simulink library "Hquad_control_LIB_MPC"  (Simulink 7.8)
settings: Solver=ode45  StartTime=0.0  StopTime=10.0  RelTol=1e-3
values from neighbouring files (symbols this model uses):
  FG_ctrl_x =     [kostas_malakies.mat]    (also in kostas_malakies2.mat)
  FG_ctrl_y =     [kostas_malakies.mat]    (also in kostas_malakies2.mat)
  FG_ctrl_yaw =     [kostas_malakies.mat]    (also in kostas_malakies2.mat)
  FG_ctrl_z =     [kostas_malakies.mat]    (also in kostas_malakies2.mat)
  g = 9.8065    [kostas_malakies.mat]    (also in kostas_malakies2.mat; load_PMModel.m = 9.81; main.m; main_last.m)
  kalm_mpc_x =     [kostas_malakies.mat]    (also in kostas_malakies2.mat)
  kalm_mpc_y =     [kostas_malakies.mat]    (also in kostas_malakies2.mat)
  kalm_mpc_yaw =     [kostas_malakies.mat]    (also in kostas_malakies2.mat)
  kalm_mpc_z =     [kostas_malakies.mat]    (also in kostas_malakies2.mat)
  MAX_BIAS_ANGLE = 0.0872664625997    [kostas_malakies.mat]    (also in kostas_malakies2.mat; main.m; main_last.m)
  MAX_BIAS_THRUST = 0.5    [kostas_malakies.mat]    (also in kostas_malakies2.mat; main.m; main_last.m)
  MAX_BIAS_YAW_RATE = 0.0872664625997    [kostas_malakies.mat]    (also in kostas_malakies2.mat; main.m; main_last.m)
  traj_FG =     [kostas.mat]    (also in kostas_malakies.mat; kostas_malakies2.mat; main_last.m = ReferenceCreator(maxdisty,maxdistz,scale_y,scale_z); traj_helix.mat)
  Ts = 0.02    [kostas_malakies.mat]    (also in kostas_malakies2.mat; main.m; main_last.m; matlab.mat = 0.08)
libraries: Hquad_control_LIB_MPC x17, simulink x9
(part 1 of 2)
settings Model: Creator=andi  LastModifiedBy=burrimi

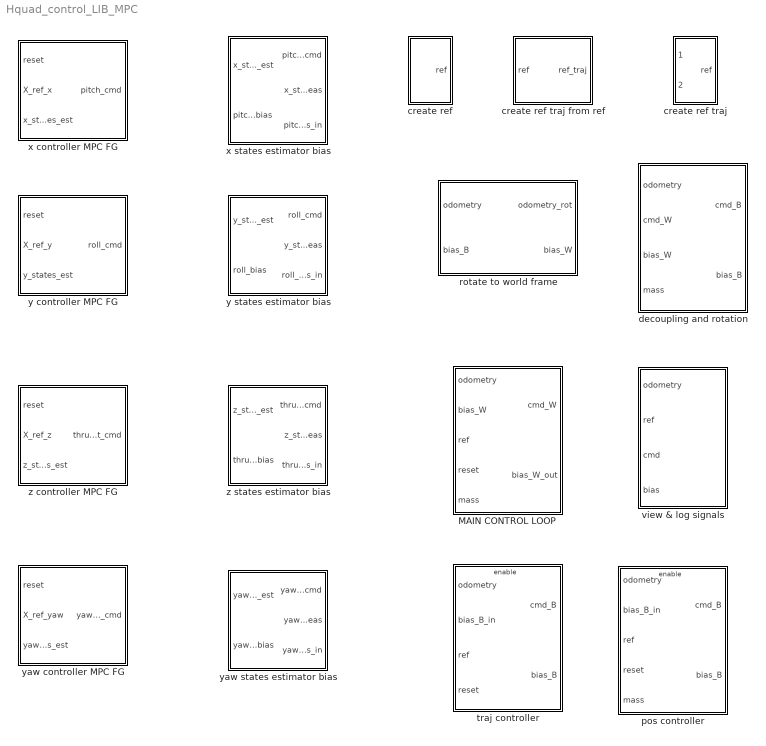
== system Hquad_control_LIB_MPC ==
  MAIN CONTROL LOOP : Subsystem  Priority=2  TreatAsAtomicUnit=on
  create ref : Subsystem
  create ref traj : Subsystem
  create ref traj from ref : Subsystem
  decoupling and rotation : Subsystem  Priority=3  TreatAsAtomicUnit=on
  pos controller : Subsystem
  rotate to world frame : Subsystem  Priority=1
  traj controller : Subsystem
  view & log signals : Subsystem
  "x controller MPC FG  " : Subsystem
  x states estimator bias : Subsystem
  y controller MPC FG : Subsystem
  y states estimator bias : Subsystem
  yaw controller MPC FG : Subsystem
  yaw states estimator bias : Subsystem
  z controller MPC FG : Subsystem
  z states estimator bias : Subsystem

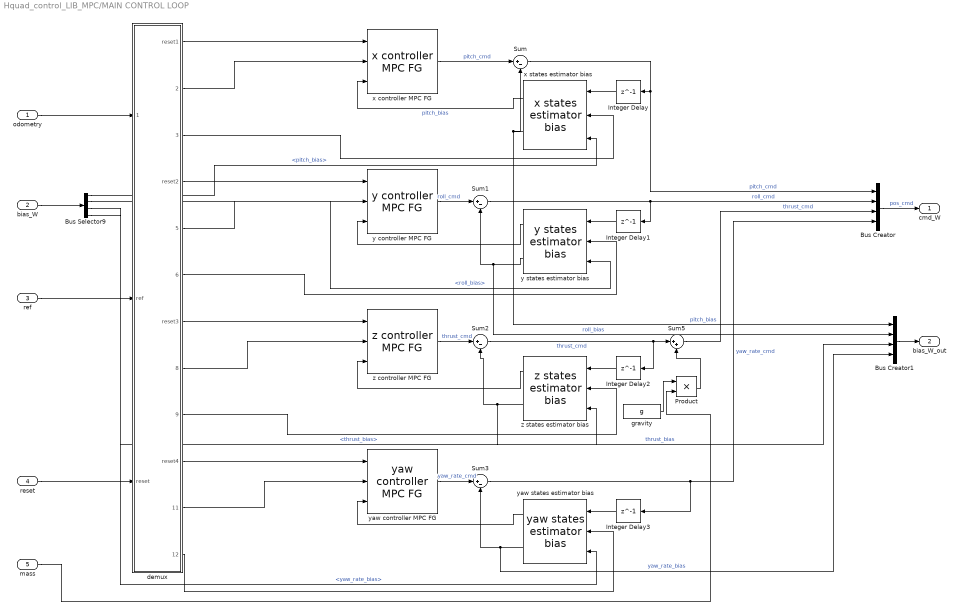
== system Hquad_control_LIB_MPC/MAIN CONTROL LOOP ==
  odometry : Inport
  bias_W : Inport  Port=2
  ref : Inport  Port=3
  reset : Inport  Port=4
  mass : Inport  Port=5
  Bus Creator : BusCreator
  Bus Creator1 : BusCreator
  Bus Selector9 : BusSelector  OutputSignals=pitch_bias,roll_bias,thrust_bias,yaw_rate_bias
  Integer Delay{,1..3} (4 alike) : Delay  DelayLength=1
  Product : Product  RndMeth=Zero
  Sum{,1..3} (4 alike) : Sum  Inputs=|+-
  Sum5 : Sum  Inputs=|++
  demux : Subsystem
  gravity : Constant  Value=g
  "x controller MPC FG  " : Hquad_control_LIB_MPC/x controller MPC FG  
  x states estimator bias : Hquad_control_LIB_MPC/x states estimator bias
  y controller MPC FG : Hquad_control_LIB_MPC/y controller MPC FG
  y states estimator bias : Hquad_control_LIB_MPC/y states estimator bias
  yaw controller MPC FG : Hquad_control_LIB_MPC/yaw controller MPC FG
  yaw states estimator bias : Hquad_control_LIB_MPC/yaw states estimator bias
  z controller MPC FG : Hquad_control_LIB_MPC/z controller MPC FG
  z states estimator bias : Hquad_control_LIB_MPC/z states estimator bias
  cmd_W : Outport
  bias_W_out : Outport  Port=2
  wires:
  gravity/1 -> Product/1
  Product/1 -> Sum5/2
  mass/1 -> Product/2
  demux/11(X_ref_yaw) -> yaw controller MPC FG/2
  demux/9(z_states_meas) -> z states estimator bias/2
  demux/6(y_states_meas) -> y states estimator bias/2
  demux/3(x_states_meas) -> x states estimator bias/2
  Bus Creator/1 -> cmd_W/1  "pos_cmd"
  demux/10(reset4) -> yaw controller MPC FG/1
  demux/7(reset3) -> z controller MPC FG/1
  demux/5(X_ref_y) -> y controller MPC FG/2
  demux/4(reset2) -> y controller MPC FG/1
  demux/1(reset1) -> "x controller MPC FG  "/1
  reset/1 -> demux/3(reset)
  ref/1 -> demux/2(ref)
  odometry/1 -> demux/1(odometry)
  Integer Delay2/1 -> z states estimator bias/1
  Integer Delay1/1 -> y states estimator bias/1
  demux/2(X_ref_x) -> "x controller MPC FG  "/2
  demux/8(X_ref_z) -> z controller MPC FG/2
  z states estimator bias/1 -> z controller MPC FG/3
  Integer Delay/1 -> x states estimator bias/1
  y states estimator bias/1 -> y controller MPC FG/3
  "x controller MPC FG  "/1 -> Sum/1  "pitch_cmd"
  Sum/1 -> Integer Delay/1, Bus Creator/1  "pitch_cmd"
  y controller MPC FG/1 -> Sum1/1  "roll_cmd"
  Sum1/1 -> Integer Delay1/1, Bus Creator/2  "roll_cmd"
  y states estimator bias/2 -> Sum1/2, Bus Creator1/2  "roll_bias"
  z states estimator bias/2 -> Sum2/2, Bus Creator1/3  "thrust_bias"
  z controller MPC FG/1 -> Sum2/1  "thrust_cmd"
  Sum2/1 -> Integer Delay2/1, Sum5/1  "thrust_cmd"
  Bus Creator1/1 -> bias_W_out/1
  Sum5/1 -> Bus Creator/3  "thrust_cmd"
  bias_W/1 -> Bus Selector9/1
  Bus Selector9/2 -> y states estimator bias/3  "<roll_bias>"
  Bus Selector9/1 -> x states estimator bias/3  "<pitch_bias>"
  demux/12(yaw_states_meas) -> yaw states estimator bias/2
  x states estimator bias/1 -> "x controller MPC FG  "/3  "pitch_bias"
  x states estimator bias/2 -> Bus Creator1/1, Sum/2  "pitch_bias"
  Bus Selector9/3 -> z states estimator bias/3  "<thrust_bias>"
  Integer Delay3/1 -> yaw states estimator bias/1
  yaw states estimator bias/1 -> yaw controller MPC FG/3
  yaw states estimator bias/2 -> Sum3/2, Bus Creator1/4  "yaw_rate_bias"
  yaw controller MPC FG/1 -> Sum3/1  "yaw_rate_cmd"
  Sum3/1 -> Bus Creator/4, Integer Delay3/1  "yaw_rate_cmd"
  Bus Selector9/4 -> yaw states estimator bias/3  "<yaw_rate_bias>"

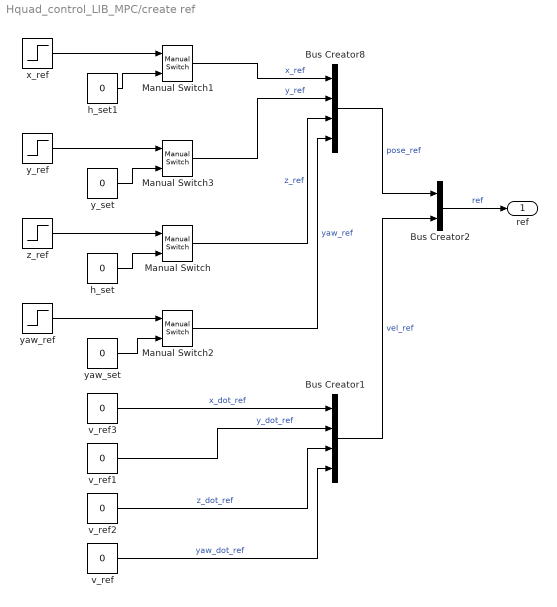
== system Hquad_control_LIB_MPC/create ref ==
  Bus Creator1 : BusCreator
  Bus Creator2 : BusCreator  Inputs=2
  Bus Creator8 : BusCreator
  Manual Switch{,1..3} (4 alike) : simulink/Signal Routing/Manual Switch  SystemSampleTime=-1  sw=1  action=0  varsize=off
  h_set : Constant  Value=0  OutDataTypeStr=double  SampleTime=-1
  h_set1 : Constant  Value=0  OutDataTypeStr=double  SampleTime=-1
  v_ref{,1..3} (4 alike) : Constant  Value=0  OutDataTypeStr=double  SampleTime=-1
  x_ref : Step  Time=5  SampleTime=0
  y_ref : Step  Time=15  SampleTime=0
  y_set : Constant  Value=0  OutDataTypeStr=double  SampleTime=-1
  yaw_ref : Step  Time=20  After=pi  SampleTime=0
  "yaw_set  " : Constant  Value=0  OutDataTypeStr=double  SampleTime=-1
  z_ref : Step  Time=15  SampleTime=0
  ref : Outport
  wires:
  yaw_ref/1 -> Manual Switch2/1
  "yaw_set  "/1 -> Manual Switch2/2
  h_set/1 -> Manual Switch/2
  z_ref/1 -> Manual Switch/1
  y_ref/1 -> Manual Switch3/1
  y_set/1 -> Manual Switch3/2
  h_set1/1 -> Manual Switch1/2
  Bus Creator2/1 -> ref/1  "ref"
  Bus Creator8/1 -> Bus Creator2/1  "pose_ref"
  Bus Creator1/1 -> Bus Creator2/2  "vel_ref"
  Manual Switch1/1 -> Bus Creator8/1  "x_ref"
  Manual Switch3/1 -> Bus Creator8/2  "y_ref"
  Manual Switch2/1 -> Bus Creator8/4  "yaw_ref"
  Manual Switch/1 -> Bus Creator8/3  "z_ref"
  v_ref/1 -> Bus Creator1/4  "yaw_dot_ref"
  v_ref3/1 -> Bus Creator1/1  "x_dot_ref"
  v_ref1/1 -> Bus Creator1/2  "y_dot_ref"
  v_ref2/1 -> Bus Creator1/3  "z_dot_ref"
  x_ref/1 -> Manual Switch1/1

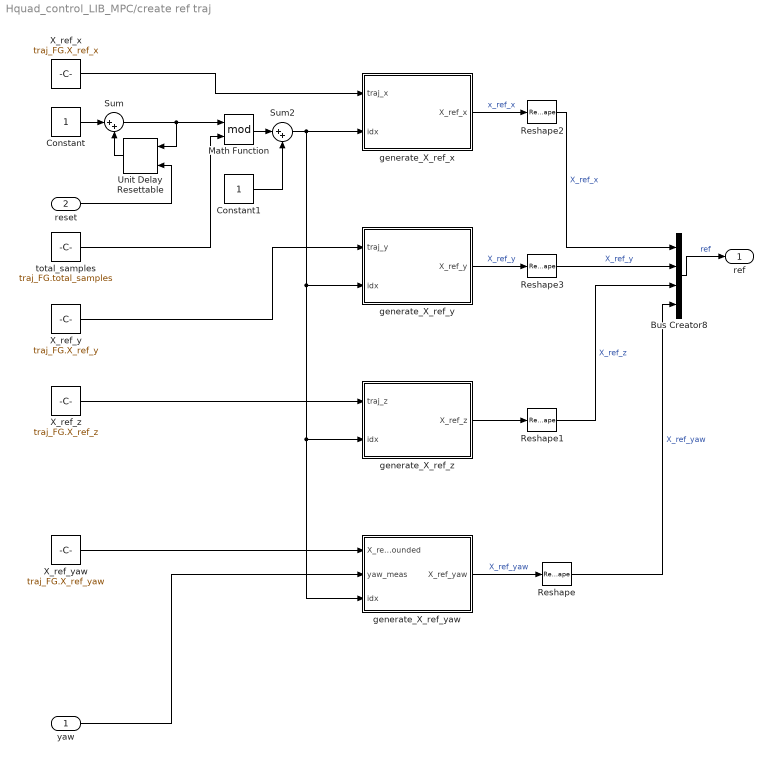
== system Hquad_control_LIB_MPC/create ref traj ==
  yaw : Inport
  reset : Inport  Port=2
  Bus Creator8 : BusCreator
  Constant : Constant
  Constant1 : Constant
  Math Function : Math  Operator=mod  SaturateOnIntegerOverflow=on
  Reshape{,1..3} (4 alike) : Reshape
  Sum : Sum  Inputs=|++
  Sum2 : Sum  Inputs=|++
  Unit Delay Resettable : simulink/Additional Math & Discrete/Additional Discrete/Unit Delay Resettable  SystemSampleTime=-1  vinit=0.0  tsamp=-1
  X_ref_x : Constant  Value=traj_FG.X_ref_x
  X_ref_y : Constant  Value=traj_FG.X_ref_y
  X_ref_yaw : Constant  Value=traj_FG.X_ref_yaw
  X_ref_z : Constant  Value=traj_FG.X_ref_z
  generate_X_ref_x : MATLAB Function  TreatAsAtomicUnit=on
  generate_X_ref_y : MATLAB Function  TreatAsAtomicUnit=on
  generate_X_ref_yaw : MATLAB Function  TreatAsAtomicUnit=on
  generate_X_ref_z : MATLAB Function  TreatAsAtomicUnit=on
  total_samples : Constant  Value=traj_FG.total_samples
  ref : Outport
  wires:
  reset/1 -> Unit Delay Resettable/2
  Bus Creator8/1 -> ref/1  "ref"
  Constant/1 -> Sum/1
  Unit Delay Resettable/1 -> Sum/2
  Sum/1 -> Unit Delay Resettable/1, Math Function/1
  total_samples/1 -> Math Function/2
  Math Function/1 -> Sum2/1
  X_ref_yaw/1 -> generate_X_ref_yaw/1(X_ref_yaw_unbounded)
  Constant1/1 -> Sum2/2
  yaw/1 -> generate_X_ref_yaw/2(yaw_meas)
  Sum2/1 -> generate_X_ref_x/2(idx), generate_X_ref_yaw/3(idx), generate_X_ref_z/2(idx), generate_X_ref_y/2(idx)
  Reshape/1 -> Bus Creator8/4  "X_ref_yaw"
  generate_X_ref_yaw/1(X_ref_yaw) -> Reshape/1  "X_ref_yaw"
  generate_X_ref_z/1(X_ref_z) -> Reshape1/1
  Reshape1/1 -> Bus Creator8/3  "X_ref_z"
  X_ref_z/1 -> generate_X_ref_z/1(traj_z)
  X_ref_y/1 -> generate_X_ref_y/1(traj_y)
  X_ref_x/1 -> generate_X_ref_x/1(traj_x)
  generate_X_ref_x/1(X_ref_x) -> Reshape2/1  "x_ref_x"
  generate_X_ref_y/1(X_ref_y) -> Reshape3/1  "X_ref_y"
  Reshape2/1 -> Bus Creator8/1  "X_ref_x"
  Reshape3/1 -> Bus Creator8/2  "X_ref_y"

== system Hquad_control_LIB_MPC/create ref traj from ref ==
  ref : Inport
  Bus Creator8 : BusCreator
  Bus Selector1 : BusSelector  OutputSignals=pose_ref.x_ref,vel_ref.x_dot_ref,pose_ref.y_ref,vel_ref.y_dot_ref,pose_ref.z_ref,vel_ref.z_dot_ref,pose_ref.yaw_ref,vel_ref.yaw_dot_ref
  generate_X_ref_x : MATLAB Function  TreatAsAtomicUnit=on
  generate_X_ref_y : MATLAB Function  TreatAsAtomicUnit=on
  generate_X_ref_yaw : MATLAB Function  TreatAsAtomicUnit=on
  generate_X_ref_z : MATLAB Function  TreatAsAtomicUnit=on
  ref_traj : Outport
  wires:
  Bus Creator8/1 -> ref_traj/1  "ref"
  generate_X_ref_x/1(X_ref) -> Bus Creator8/1  "X_ref_x"
  generate_X_ref_y/1(X_ref) -> Bus Creator8/2  "X_ref_y"
  generate_X_ref_z/1(X_ref) -> Bus Creator8/3  "X_ref_z"
  generate_X_ref_yaw/1(X_ref) -> Bus Creator8/4  "X_ref_yaw"
  ref/1 -> Bus Selector1/1
  Bus Selector1/1 -> generate_X_ref_x/1(x_ref)  "<x_ref>"
  Bus Selector1/2 -> generate_X_ref_x/2(x_dot_ref)  "<x_dot_ref>"
  Bus Selector1/3 -> generate_X_ref_y/1(x_ref)  "<y_ref>"
  Bus Selector1/4 -> generate_X_ref_y/2(x_dot_ref)  "<y_dot_ref>"
  Bus Selector1/5 -> generate_X_ref_z/1(x_ref)  "<z_ref>"
  Bus Selector1/6 -> generate_X_ref_z/2(x_dot_ref)  "<z_dot_ref>"
  Bus Selector1/7 -> generate_X_ref_yaw/1(x_ref)  "<yaw_ref>"
  Bus Selector1/8 -> generate_X_ref_yaw/2(x_dot_ref)  "<yaw_dot_ref>"

== system Hquad_control_LIB_MPC/decoupling and rotation ==
  note: 
  odometry : Inport
  cmd_W : Inport  Port=2
  bias_W : Inport  Port=3
  mass : Inport  Port=4
  Bus Selector1 : BusSelector  OutputSignals=rpy.yaw
  Bus Selector2 : BusSelector  OutputSignals=rpy.roll,rpy.pitch
  "decoupling " : Subsystem
  rotate_to_quat_frame : Subsystem
  cmd_B : Outport
  bias_B : Outport  Port=2
  wires:
  mass/1 -> "decoupling "/4(mass)
  rotate_to_quat_frame/1("cmd_rot  ") -> cmd_B/1  "roll_cmd"
  "decoupling "/1("cmd_comp  ") -> rotate_to_quat_frame/2(cmd_comp)  "thrust_cmd"
  odometry/1 -> Bus Selector1/1, Bus Selector2/1
  Bus Selector1/1 -> rotate_to_quat_frame/1(yaw_meas)  "<yaw>"
  rotate_to_quat_frame/2(bias_rot) -> bias_B/1
  bias_W/1 -> rotate_to_quat_frame/3(bias)
  cmd_W/1 -> "decoupling "/3(cmd)
  Bus Selector2/1 -> "decoupling "/1("roll_meas  ")  "<roll>"
  Bus Selector2/2 -> "decoupling "/2("pitch_meas  ")  "<pitch>"

== system Hquad_control_LIB_MPC/pos controller ==
  odometry : Inport
  bias_B_in : Inport  Port=2
  ref : Inport  Port=3
  reset : Inport  Port=4
  mass : Inport  Port=5
  Enable : EnablePort  StatesWhenEnabling=reset
  MAIN CONTROL LOOP1 : Hquad_control_LIB_MPC/MAIN CONTROL LOOP  Priority=2
  decoupling and rotation : Hquad_control_LIB_MPC/decoupling and rotation  Priority=3
  get ref from vector : Subsystem
  mode1 : Scope
      settings: YMin=0  YMax=6  SaveName=ScopeData12
  rotate to world frame : Hquad_control_LIB_MPC/rotate to world frame  Priority=1
  view & log signals : Hquad_control_LIB_MPC/view & log signals
  cmd_B : Outport
  bias_B : Outport  Port=2
  wires:
  mass/1 -> decoupling and rotation/4, MAIN CONTROL LOOP1/5
  bias_B_in/1 -> rotate to world frame/2
  rotate to world frame/2 -> MAIN CONTROL LOOP1/2
  decoupling and rotation/2 -> bias_B/1
  decoupling and rotation/1 -> cmd_B/1
  MAIN CONTROL LOOP1/2 -> view & log signals/4, decoupling and rotation/3
  rotate to world frame/1 -> decoupling and rotation/1, MAIN CONTROL LOOP1/1
  get ref from vector/1(ref) -> mode1/1, view & log signals/2
  ref/1 -> MAIN CONTROL LOOP1/3, get ref from vector/1(X_ref)
  reset/1 -> MAIN CONTROL LOOP1/4
  odometry/1 -> view & log signals/1, rotate to world frame/1
  MAIN CONTROL LOOP1/1 -> view & log signals/3, decoupling and rotation/2

== system Hquad_control_LIB_MPC/rotate to world frame ==
  odometry : Inport
  bias_B : Inport  Port=2
  Bus Creator1 : BusCreator  Inputs=3
  Bus Creator2 : BusCreator
  Bus Creator5 : BusCreator
  Bus Selector1 : BusSelector  OutputSignals=rpy.roll,rpy.pitch
  Bus Selector2 : BusSelector  OutputSignals=ang_vel
  Bus Selector3 : BusSelector  OutputSignals=rpy.yaw
  Bus Selector4 : BusSelector  OutputSignals=thrust_bias,yaw_rate_bias
  Bus Selector5 : BusSelector  OutputSignals=pitch_bias,roll_bias
  Bus Selector6 : BusSelector  OutputSignals=pos,vel
  Embedded MATLAB Function : MATLAB Function  TreatAsAtomicUnit=on
  odometry_rot : Outport
  bias_W : Outport  Port=2
  wires:
  Bus Selector6/2 -> Bus Creator5/2  "<vel>"
  Bus Selector6/1 -> Bus Creator5/1  "<pos>"
  Bus Creator5/1 -> odometry_rot/1  "odom"
  Bus Selector3/1 -> Embedded MATLAB Function/5(yaw), Bus Creator1/3  "<yaw>"
  odometry/1 -> Bus Selector3/1, Bus Selector1/1, Bus Selector6/1, Bus Selector2/1
  Bus Selector2/1 -> Bus Creator5/4  "<ang_vel>"
  Bus Creator1/1 -> Bus Creator5/3  "rpy"
  Embedded MATLAB Function/1(roll_rot) -> Bus Creator1/1  "roll"
  Embedded MATLAB Function/2(pitch_rot) -> Bus Creator1/2  "pitch"
  Bus Selector1/1 -> Embedded MATLAB Function/1(roll)  "<roll>"
  Bus Selector1/2 -> Embedded MATLAB Function/2(pitch)  "<pitch>"
  Bus Creator2/1 -> bias_W/1
  Bus Selector4/2 -> Bus Creator2/4  "<yaw_rate_bias>"
  Bus Selector4/1 -> Bus Creator2/3  "<thrust_bias>"
  Bus Selector5/1 -> Embedded MATLAB Function/3(pitch_bias)  "<pitch_bias>"
  Bus Selector5/2 -> Embedded MATLAB Function/4(roll_bias)  "<roll_bias>"
  bias_B/1 -> Bus Selector5/1, Bus Selector4/1
  Embedded MATLAB Function/3(pitch_bias_rot) -> Bus Creator2/1  "pitch_bias"
  Embedded MATLAB Function/4(roll_bias_rot) -> Bus Creator2/2  "roll_bias"

== system Hquad_control_LIB_MPC/traj controller ==
  odometry : Inport
  bias_B_in : Inport  Port=2
  ref : Inport  Port=3
  reset : Inport  Port=4
  Enable : EnablePort  StatesWhenEnabling=reset
  Bus Selector9 : BusSelector  OutputSignals=rpy.yaw
  MAIN CONTROL LOOP1 : Hquad_control_LIB_MPC/MAIN CONTROL LOOP  Priority=2  SystemSampleTime=-1
  Terminator : Terminator
  create ref traj : Hquad_control_LIB_MPC/create ref traj  SystemSampleTime=-1
  decoupling and rotation : Hquad_control_LIB_MPC/decoupling and rotation  Priority=3  SystemSampleTime=-1
  get ref from vector : Subsystem
  rotate to world frame : Hquad_control_LIB_MPC/rotate to world frame  Priority=1  SystemSampleTime=-1
  view & log signals : Hquad_control_LIB_MPC/view & log signals  SystemSampleTime=-1
  cmd_B : Outport
  bias_B : Outport  Port=2
  wires:
  ref/1 -> Terminator/1
  Bus Selector9/1 -> create ref traj/1  "<yaw>"
  bias_B_in/1 -> rotate to world frame/2
  rotate to world frame/2 -> MAIN CONTROL LOOP1/2
  decoupling and rotation/2 -> bias_B/1
  decoupling and rotation/1 -> cmd_B/1
  MAIN CONTROL LOOP1/2 -> decoupling and rotation/3, view & log signals/4
  rotate to world frame/1 -> decoupling and rotation/1, MAIN CONTROL LOOP1/1
  get ref from vector/1(ref) -> view & log signals/2
  reset/1 -> create ref traj/2, MAIN CONTROL LOOP1/4
  odometry/1 -> rotate to world frame/1, view & log signals/1, Bus Selector9/1
  MAIN CONTROL LOOP1/1 -> decoupling and rotation/2, view & log signals/3
  create ref traj/1 -> get ref from vector/1(X_ref), MAIN CONTROL LOOP1/3

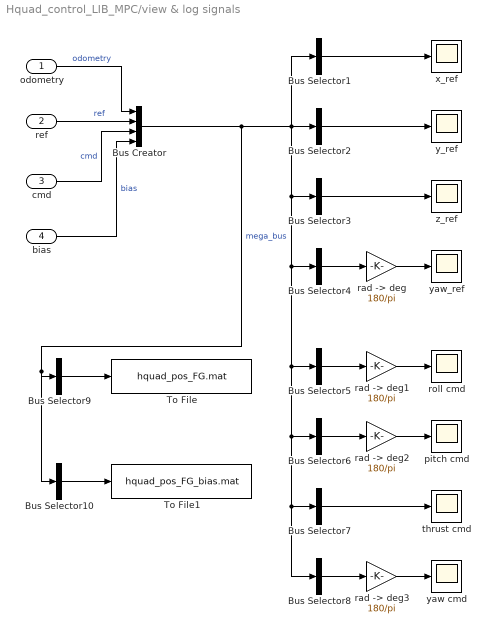
== system Hquad_control_LIB_MPC/view & log signals ==
  odometry : Inport
  ref : Inport  Port=2
  cmd : Inport  Port=3
  bias : Inport  Port=4
  Bus Creator : BusCreator
  Bus Selector1 : BusSelector  OutputSignals=odometry.pos.x,odometry.vel.x_dot,ref.pose_ref.x_ref,ref.vel_ref.x_dot_ref  OutputAsBus=on
  Bus Selector10 : BusSelector  OutputSignals=bias.pitch_bias,bias.roll_bias,bias.thrust_bias,bias.yaw_rate_bias  OutputAsBus=on
  Bus Selector2 : BusSelector  OutputSignals=odometry.pos.y,odometry.vel.y_dot,ref.pose_ref.y_ref,ref.vel_ref.y_dot_ref  OutputAsBus=on
  Bus Selector3 : BusSelector  OutputSignals=odometry.pos.z,odometry.vel.z_dot,ref.pose_ref.z_ref,ref.vel_ref.z_dot_ref  OutputAsBus=on
  Bus Selector4 : BusSelector  OutputSignals=odometry.rpy.yaw,odometry.ang_vel.ang_vel_z,ref.pose_ref.yaw_ref,ref.vel_ref.yaw_dot_ref  OutputAsBus=on
  Bus Selector5 : BusSelector  OutputSignals=odometry.rpy.roll,odometry.ang_vel.ang_vel_x,cmd.roll_cmd  OutputAsBus=on
  Bus Selector6 : BusSelector  OutputSignals=odometry.rpy.pitch,odometry.ang_vel.ang_vel_y,cmd.pitch_cmd  OutputAsBus=on
  Bus Selector7 : BusSelector  OutputSignals=odometry.pos.z,ref.pose_ref.z_ref,cmd.thrust_cmd  OutputAsBus=on
  Bus Selector8 : BusSelector  OutputSignals=odometry.rpy.yaw,odometry.ang_vel.ang_vel_z,cmd.yaw_rate_cmd  OutputAsBus=on
  Bus Selector9 : BusSelector  OutputSignals=odometry.pos.x,odometry.vel.x_dot,odometry.rpy.pitch,ref.pose_ref.x_ref,cmd.pitch_cmd,odometry.pos.y,odometry.vel.y_dot,odometry.rpy.roll,ref.pose_ref.y_ref,cmd.roll_cmd,odometry.pos.z,odometry.vel.z_dot,ref.pose_ref.z_ref,cmd.thrust_cmd,odometry.rpy.yaw,odometry.ang_vel.ang_vel_z,ref.pose_ref.yaw_ref,cmd.yaw_rate_cmd  OutputAsBus=on
  To File : ToFile  Filename=hquad_pos_FG.mat  MatrixName=hquad_pos_FG
  To File1 : ToFile  Filename=hquad_pos_FG_bias.mat  MatrixName=hquad_pos_FG_bias
  pitch cmd : Scope
      settings: YMin=-15  YMax=15  SaveName=ScopeData2
  rad -> deg{,1..3} (4 alike) : Gain  Gain=180/pi
  roll cmd : Scope
      settings: YMin=-100  YMax=100
  thrust cmd : Scope
      settings: YMin=-3  YMax=3  SaveName=ScopeData11
  x_ref : Scope
      settings: YMin=-1.5  YMax=1.5  SaveName=ScopeData3
  y_ref : Scope
      settings: TimeRange=40  YMin=-0.75  YMax=2.75
  yaw cmd : Scope
      settings: YMin=-60  YMax=60  SaveName=ScopeData10
  yaw_ref : Scope
      settings: TimeRange=39.996  YMin=-190  YMax=190  SaveName=ScopeData8
  z_ref : Scope
      settings: TimeRange=40  YMin=-21  YMax=1  SaveName=ScopeData5
  wires:
  Bus Selector9/1 -> To File/1
  Bus Selector10/1 -> To File1/1
  "rad -> deg"/1 -> yaw_ref/1
  "rad -> deg1"/1 -> roll cmd/1
  "rad -> deg2"/1 -> pitch cmd/1
  "rad -> deg3"/1 -> yaw cmd/1
  odometry/1 -> Bus Creator/1  "odometry"
  ref/1 -> Bus Creator/2  "ref"
  cmd/1 -> Bus Creator/3  "cmd"
  Bus Creator/1 -> Bus Selector9/1, Bus Selector10/1, Bus Selector1/1, Bus Selector2/1, Bus Selector3/1, Bus Selector4/1, Bus Selector5/1, Bus Selector6/1, Bus Selector7/1, Bus Selector8/1  "mega_bus"
  Bus Selector1/1 -> x_ref/1
  Bus Selector2/1 -> y_ref/1
  Bus Selector3/1 -> z_ref/1
  Bus Selector4/1 -> "rad -> deg"/1
  Bus Selector7/1 -> thrust cmd/1
  Bus Selector5/1 -> "rad -> deg1"/1
  Bus Selector6/1 -> "rad -> deg2"/1
  Bus Selector8/1 -> "rad -> deg3"/1
  bias/1 -> Bus Creator/4  "bias"

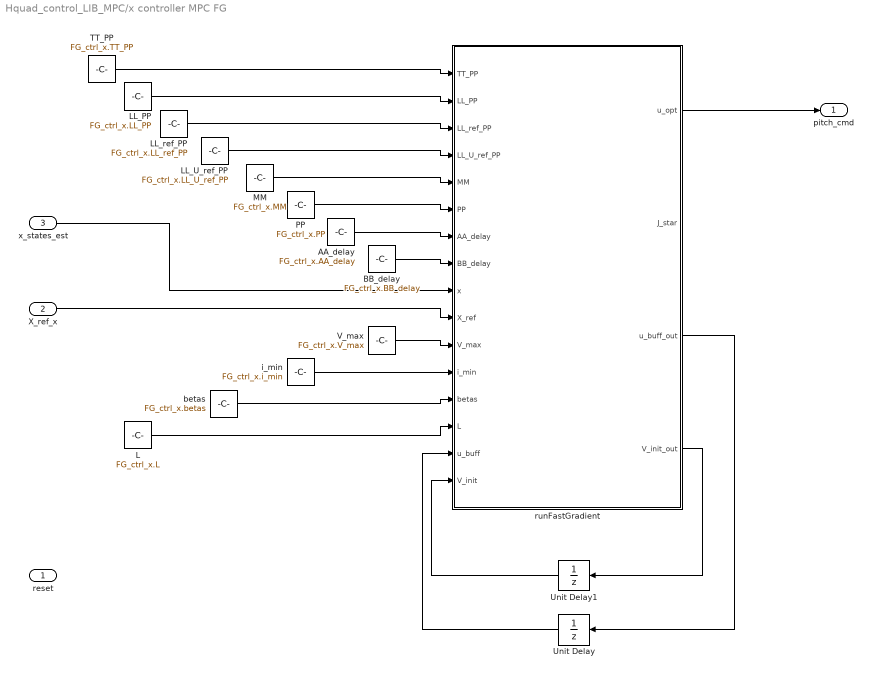
== system Hquad_control_LIB_MPC/x controller MPC FG   ==
  reset : Inport  PortDimensions=1
  "X_ref_x  " : Inport  Port=2
  "x_states_est  " : Inport  Port=3
  AA_delay : Constant  Value=FG_ctrl_x.AA_delay
  BB_delay : Constant  Value=FG_ctrl_x.BB_delay
  L : Constant  Value=FG_ctrl_x.L
  LL_PP : Constant  Value=FG_ctrl_x.LL_PP
  LL_U_ref_PP : Constant  Value=FG_ctrl_x.LL_U_ref_PP
  LL_ref_PP : Constant  Value=FG_ctrl_x.LL_ref_PP
  MM : Constant  Value=FG_ctrl_x.MM
  PP : Constant  Value=FG_ctrl_x.PP
  TT_PP : Constant  Value=FG_ctrl_x.TT_PP
  Unit Delay : UnitDelay  X0=zeros(FG_ctrl_x.delay_steps,1)  SampleTime=-1
  Unit Delay1 : UnitDelay  X0=zeros(size(FG_ctrl_x.V_max,1),1)  SampleTime=-1
  V_max : Constant  Value=FG_ctrl_x.V_max
  betas : Constant  Value=FG_ctrl_x.betas
  i_min : Constant  Value=FG_ctrl_x.i_min
  runFastGradient : MATLAB Function  TreatAsAtomicUnit=on
  "pitch_cmd   " : Outport  PortDimensions=1
  wires:
  "x_states_est  "/1 -> runFastGradient/9(x)
  runFastGradient/1(u_opt) -> "pitch_cmd   "/1
  "X_ref_x  "/1 -> runFastGradient/10(X_ref)
  TT_PP/1 -> runFastGradient/1(TT_PP)
  LL_PP/1 -> runFastGradient/2(LL_PP)
  runFastGradient/4(V_init_out) -> Unit Delay1/1
  runFastGradient/3(u_buff_out) -> Unit Delay/1
  Unit Delay1/1 -> runFastGradient/16(V_init)
  Unit Delay/1 -> runFastGradient/15(u_buff)
  LL_ref_PP/1 -> runFastGradient/3(LL_ref_PP)
  MM/1 -> runFastGradient/5(MM)
  PP/1 -> runFastGradient/6(PP)
  AA_delay/1 -> runFastGradient/7(AA_delay)
  BB_delay/1 -> runFastGradient/8(BB_delay)
  V_max/1 -> runFastGradient/11(V_max)
  i_min/1 -> runFastGradient/12(i_min)
  betas/1 -> runFastGradient/13(betas)
  L/1 -> runFastGradient/14(L)
  LL_U_ref_PP/1 -> runFastGradient/4(LL_U_ref_PP)

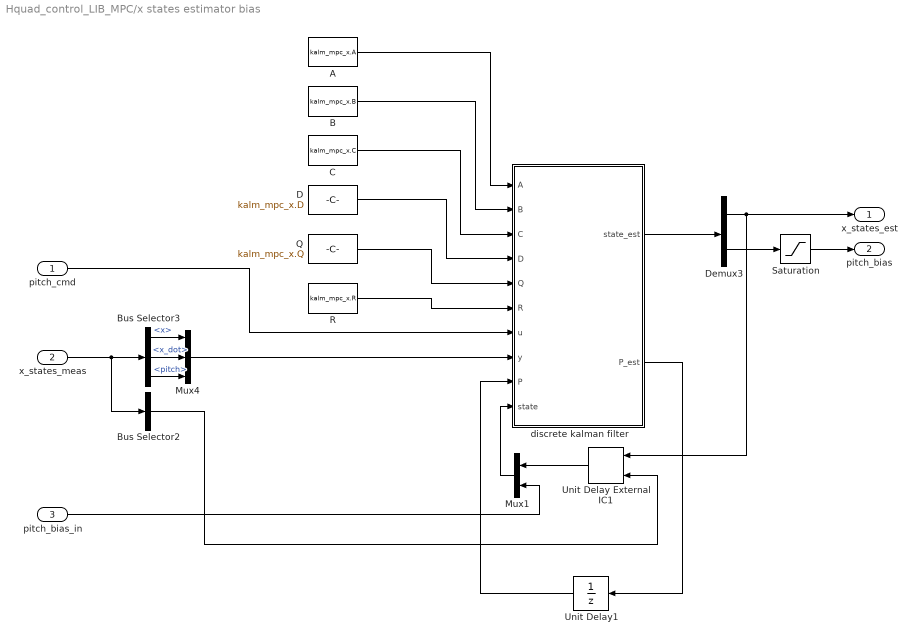
== system Hquad_control_LIB_MPC/x states estimator bias ==
  pitch_cmd : Inport  PortDimensions=1
  x_states_meas : Inport  Port=2  PortDimensions=3
  pitch_bias_in : Inport  Port=3  PortDimensions=1
  A : Constant  Value=kalm_mpc_x.A
  B : Constant  Value=kalm_mpc_x.B
  Bus Selector2 : BusSelector  OutputSignals=x,x_dot,pitch  OutputAsBus=on
  Bus Selector3 : BusSelector  OutputSignals=x,x_dot,pitch
  C : Constant  Value=kalm_mpc_x.C
  D : Constant  Value=kalm_mpc_x.D
  Demux3 : Demux  Outputs=2
  Mux1 : Mux  Inputs=2
  Mux4 : Mux  Inputs=3
  Q : Constant  Value=kalm_mpc_x.Q
  R : Constant  Value=kalm_mpc_x.R
  Saturation : Saturate  UpperLimit=MAX_BIAS_ANGLE  LowerLimit=-MAX_BIAS_ANGLE
  Unit Delay External IC1 : simulink/Additional Math & Discrete/Additional Discrete/Unit Delay External IC  SystemSampleTime=-1  tsamp=-1
  Unit Delay1 : UnitDelay  X0=kalm_mpc_x.P  SampleTime=Ts
  discrete kalman filter : MATLAB Function  AncestorBlock=Hquad_control_LIB_LQRI/x states estimator/discrete kalman filter  TreatAsAtomicUnit=on
  x_states_est : Outport  PortDimensions=3
  pitch_bias : Outport  Port=2  PortDimensions=1
  wires:
  x_states_meas/1 -> Bus Selector3/1, Bus Selector2/1
  Bus Selector2/1 -> Unit Delay External IC1/2
  A/1 -> discrete kalman filter/1(A)
  B/1 -> discrete kalman filter/2(B)
  C/1 -> discrete kalman filter/3(C)
  D/1 -> discrete kalman filter/4(D)
  discrete kalman filter/1(state_est) -> Demux3/1
  discrete kalman filter/2(P_est) -> Unit Delay1/1
  Unit Delay1/1 -> discrete kalman filter/9(P)
  pitch_cmd/1 -> discrete kalman filter/7(u)
  Bus Selector3/1 -> Mux4/1  "<x>"
  Bus Selector3/2 -> Mux4/2  "<x_dot>"
  Bus Selector3/3 -> Mux4/3  "<pitch>"
  Mux4/1 -> discrete kalman filter/8(y)
  Q/1 -> discrete kalman filter/5(Q)
  R/1 -> discrete kalman filter/6(R)
  Demux3/2 -> Saturation/1
  Demux3/1 -> x_states_est/1, Unit Delay External IC1/1
  Saturation/1 -> pitch_bias/1
  Mux1/1 -> discrete kalman filter/10(state)
  pitch_bias_in/1 -> Mux1/2
  Unit Delay External IC1/1 -> Mux1/1

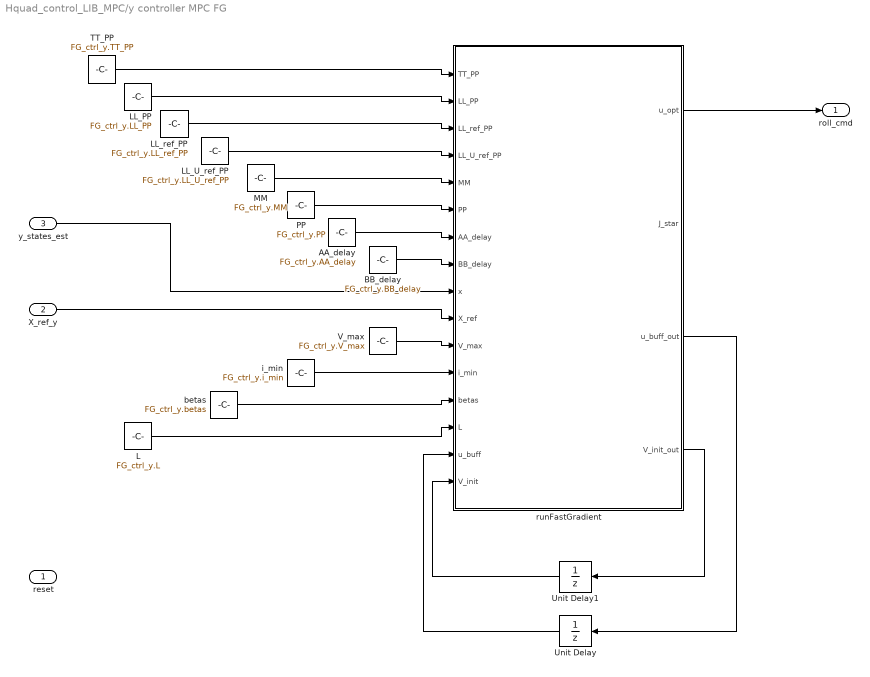
== system Hquad_control_LIB_MPC/y controller MPC FG ==
  reset : Inport  PortDimensions=1
  "X_ref_y  " : Inport  Port=2
  "y_states_est  " : Inport  Port=3
  AA_delay : Constant  Value=FG_ctrl_y.AA_delay
  BB_delay : Constant  Value=FG_ctrl_y.BB_delay
  L : Constant  Value=FG_ctrl_y.L
  LL_PP : Constant  Value=FG_ctrl_y.LL_PP
  LL_U_ref_PP : Constant  Value=FG_ctrl_y.LL_U_ref_PP
  LL_ref_PP : Constant  Value=FG_ctrl_y.LL_ref_PP
  MM : Constant  Value=FG_ctrl_y.MM
  PP : Constant  Value=FG_ctrl_y.PP
  TT_PP : Constant  Value=FG_ctrl_y.TT_PP
  Unit Delay : UnitDelay  X0=zeros(FG_ctrl_y.delay_steps,1)  SampleTime=-1
  Unit Delay1 : UnitDelay  X0=zeros(size(FG_ctrl_y.V_max,1),1)  SampleTime=-1
  V_max : Constant  Value=FG_ctrl_y.V_max
  betas : Constant  Value=FG_ctrl_y.betas
  i_min : Constant  Value=FG_ctrl_y.i_min
  runFastGradient : MATLAB Function  TreatAsAtomicUnit=on
  roll_cmd : Outport  PortDimensions=1
  wires:
  "y_states_est  "/1 -> runFastGradient/9(x)
  runFastGradient/1(u_opt) -> roll_cmd/1
  "X_ref_y  "/1 -> runFastGradient/10(X_ref)
  TT_PP/1 -> runFastGradient/1(TT_PP)
  LL_PP/1 -> runFastGradient/2(LL_PP)
  runFastGradient/4(V_init_out) -> Unit Delay1/1
  runFastGradient/3(u_buff_out) -> Unit Delay/1
  Unit Delay1/1 -> runFastGradient/16(V_init)
  Unit Delay/1 -> runFastGradient/15(u_buff)
  LL_ref_PP/1 -> runFastGradient/3(LL_ref_PP)
  MM/1 -> runFastGradient/5(MM)
  PP/1 -> runFastGradient/6(PP)
  AA_delay/1 -> runFastGradient/7(AA_delay)
  BB_delay/1 -> runFastGradient/8(BB_delay)
  V_max/1 -> runFastGradient/11(V_max)
  i_min/1 -> runFastGradient/12(i_min)
  betas/1 -> runFastGradient/13(betas)
  L/1 -> runFastGradient/14(L)
  LL_U_ref_PP/1 -> runFastGradient/4(LL_U_ref_PP)

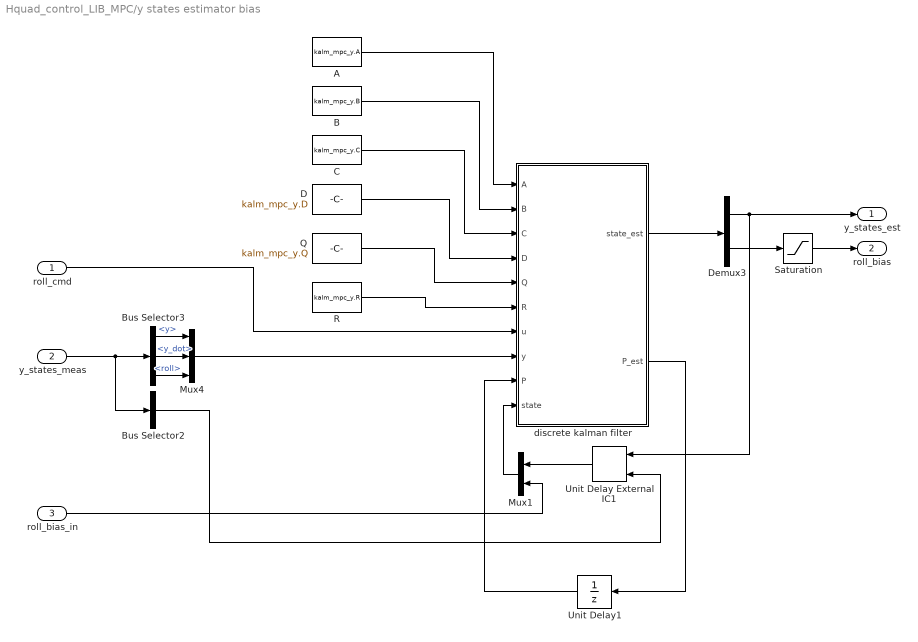
== system Hquad_control_LIB_MPC/y states estimator bias ==
  roll_cmd : Inport  PortDimensions=1
  y_states_meas : Inport  Port=2  PortDimensions=3
  roll_bias_in : Inport  Port=3  PortDimensions=1
  A : Constant  Value=kalm_mpc_y.A
  B : Constant  Value=kalm_mpc_y.B
  Bus Selector2 : BusSelector  OutputSignals=y,y_dot,roll  OutputAsBus=on
  Bus Selector3 : BusSelector  OutputSignals=y,y_dot,roll
  C : Constant  Value=kalm_mpc_y.C
  D : Constant  Value=kalm_mpc_y.D
  Demux3 : Demux  Outputs=2
  Mux1 : Mux  Inputs=2
  Mux4 : Mux  Inputs=3
  Q : Constant  Value=kalm_mpc_y.Q
  R : Constant  Value=kalm_mpc_y.R
  Saturation : Saturate  UpperLimit=MAX_BIAS_ANGLE  LowerLimit=-MAX_BIAS_ANGLE
  Unit Delay External IC1 : simulink/Additional Math & Discrete/Additional Discrete/Unit Delay External IC  SystemSampleTime=-1  tsamp=-1
  Unit Delay1 : UnitDelay  X0=kalm_mpc_y.P  SampleTime=Ts
  discrete kalman filter : MATLAB Function  AncestorBlock=Hquad_control_LIB_LQRI/x states estimator/discrete kalman filter  TreatAsAtomicUnit=on
  y_states_est : Outport  PortDimensions=3
  roll_bias : Outport  Port=2  PortDimensions=1
  wires:
  y_states_meas/1 -> Bus Selector3/1, Bus Selector2/1
  Bus Selector2/1 -> Unit Delay External IC1/2
  A/1 -> discrete kalman filter/1(A)
  B/1 -> discrete kalman filter/2(B)
  C/1 -> discrete kalman filter/3(C)
  D/1 -> discrete kalman filter/4(D)
  discrete kalman filter/1(state_est) -> Demux3/1
  discrete kalman filter/2(P_est) -> Unit Delay1/1
  Unit Delay1/1 -> discrete kalman filter/9(P)
  roll_cmd/1 -> discrete kalman filter/7(u)
  Bus Selector3/1 -> Mux4/1  "<y>"
  Bus Selector3/2 -> Mux4/2  "<y_dot>"
  Bus Selector3/3 -> Mux4/3  "<roll>"
  Mux4/1 -> discrete kalman filter/8(y)
  Q/1 -> discrete kalman filter/5(Q)
  R/1 -> discrete kalman filter/6(R)
  Demux3/2 -> Saturation/1
  Demux3/1 -> Unit Delay External IC1/1, y_states_est/1
  Saturation/1 -> roll_bias/1
  Mux1/1 -> discrete kalman filter/10(state)
  roll_bias_in/1 -> Mux1/2
  Unit Delay External IC1/1 -> Mux1/1

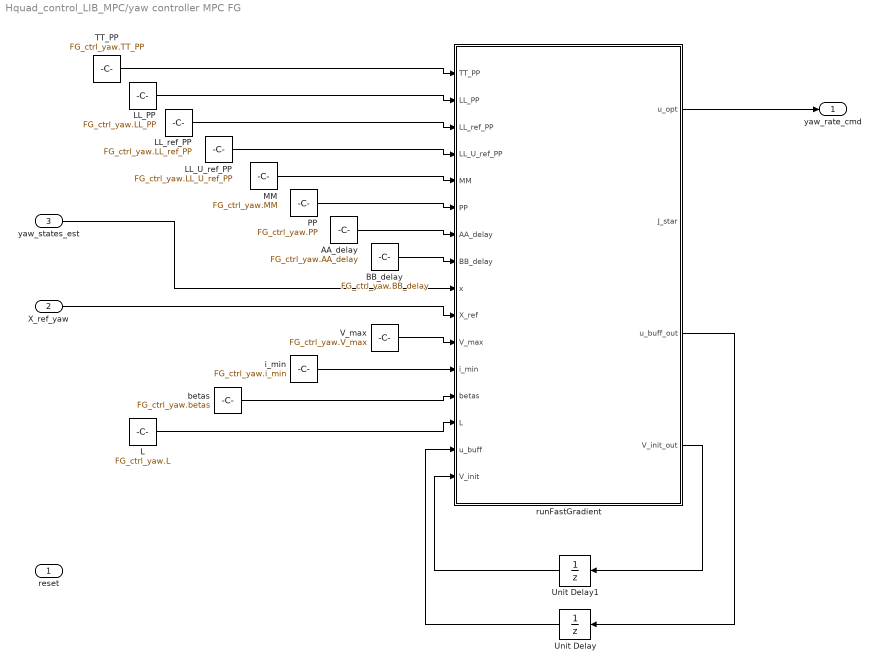
== system Hquad_control_LIB_MPC/yaw controller MPC FG ==
  reset : Inport  PortDimensions=1
  X_ref_yaw : Inport  Port=2
  "yaw_states_est  " : Inport  Port=3
  AA_delay : Constant  Value=FG_ctrl_yaw.AA_delay
  BB_delay : Constant  Value=FG_ctrl_yaw.BB_delay
  L : Constant  Value=FG_ctrl_yaw.L
  LL_PP : Constant  Value=FG_ctrl_yaw.LL_PP
  LL_U_ref_PP : Constant  Value=FG_ctrl_yaw.LL_U_ref_PP
  LL_ref_PP : Constant  Value=FG_ctrl_yaw.LL_ref_PP
  MM : Constant  Value=FG_ctrl_yaw.MM
  PP : Constant  Value=FG_ctrl_yaw.PP
  TT_PP : Constant  Value=FG_ctrl_yaw.TT_PP
  Unit Delay : UnitDelay  X0=zeros(FG_ctrl_yaw.delay_steps,1)  SampleTime=-1
  Unit Delay1 : UnitDelay  X0=zeros(size(FG_ctrl_yaw.V_max,1),1)  SampleTime=-1
  V_max : Constant  Value=FG_ctrl_yaw.V_max
  betas : Constant  Value=FG_ctrl_yaw.betas
  i_min : Constant  Value=FG_ctrl_yaw.i_min
  runFastGradient : MATLAB Function  TreatAsAtomicUnit=on
  yaw_rate_cmd : Outport  PortDimensions=1
  wires:
  "yaw_states_est  "/1 -> runFastGradient/9(x)
  runFastGradient/1(u_opt) -> yaw_rate_cmd/1
  X_ref_yaw/1 -> runFastGradient/10(X_ref)
  TT_PP/1 -> runFastGradient/1(TT_PP)
  LL_PP/1 -> runFastGradient/2(LL_PP)
  runFastGradient/4(V_init_out) -> Unit Delay1/1
  runFastGradient/3(u_buff_out) -> Unit Delay/1
  Unit Delay1/1 -> runFastGradient/16(V_init)
  Unit Delay/1 -> runFastGradient/15(u_buff)
  LL_ref_PP/1 -> runFastGradient/3(LL_ref_PP)
  MM/1 -> runFastGradient/5(MM)
  PP/1 -> runFastGradient/6(PP)
  AA_delay/1 -> runFastGradient/7(AA_delay)
  BB_delay/1 -> runFastGradient/8(BB_delay)
  V_max/1 -> runFastGradient/11(V_max)
  i_min/1 -> runFastGradient/12(i_min)
  betas/1 -> runFastGradient/13(betas)
  L/1 -> runFastGradient/14(L)
  LL_U_ref_PP/1 -> runFastGradient/4(LL_U_ref_PP)

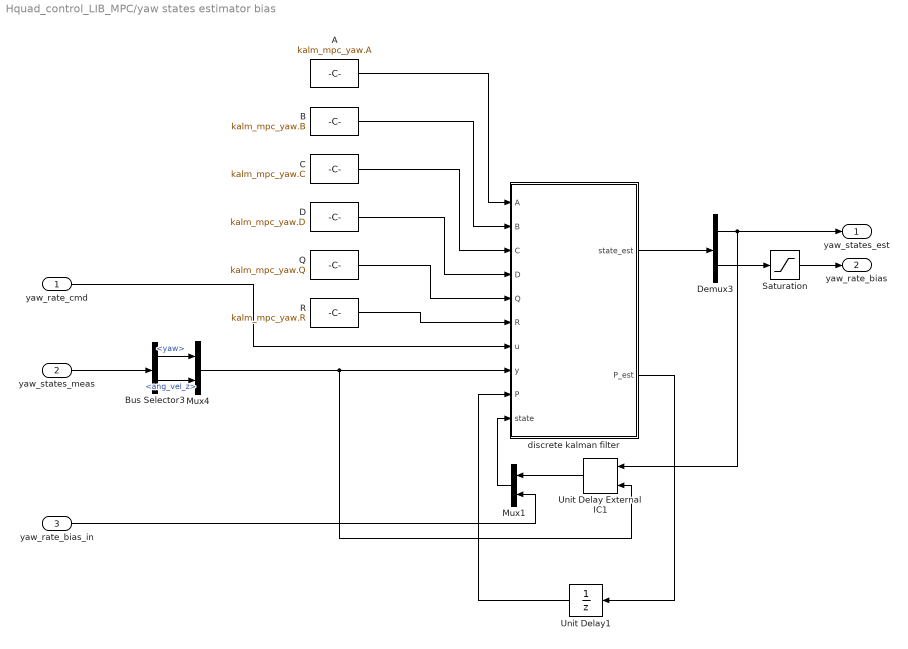
== system Hquad_control_LIB_MPC/yaw states estimator bias ==
  yaw_rate_cmd : Inport  PortDimensions=1
  yaw_states_meas : Inport  Port=2  PortDimensions=2
  yaw_rate_bias_in : Inport  Port=3  PortDimensions=1
  A : Constant  Value=kalm_mpc_yaw.A
  B : Constant  Value=kalm_mpc_yaw.B
  Bus Selector3 : BusSelector  OutputSignals=yaw,ang_vel_z
  C : Constant  Value=kalm_mpc_yaw.C
  D : Constant  Value=kalm_mpc_yaw.D
  Demux3 : Demux  Outputs=2
  Mux1 : Mux  Inputs=2
  Mux4 : Mux  Inputs=2
  Q : Constant  Value=kalm_mpc_yaw.Q
  R : Constant  Value=kalm_mpc_yaw.R
  Saturation : Saturate  UpperLimit=MAX_BIAS_YAW_RATE  LowerLimit=-MAX_BIAS_YAW_RATE
  Unit Delay External IC1 : simulink/Additional Math & Discrete/Additional Discrete/Unit Delay External IC  SystemSampleTime=-1  tsamp=-1
  Unit Delay1 : UnitDelay  X0=kalm_mpc_yaw.P  SampleTime=Ts
  discrete kalman filter : MATLAB Function  AncestorBlock=Hquad_control_LIB_LQRI/x states estimator/discrete kalman filter  TreatAsAtomicUnit=on
  yaw_states_est : Outport  PortDimensions=2
  yaw_rate_bias : Outport  Port=2  PortDimensions=1
  wires:
  Bus Selector3/2 -> Mux4/2  "<ang_vel_z>"
  Bus Selector3/1 -> Mux4/1  "<yaw>"
  yaw_states_meas/1 -> Bus Selector3/1
  A/1 -> discrete kalman filter/1(A)
  B/1 -> discrete kalman filter/2(B)
  C/1 -> discrete kalman filter/3(C)
  D/1 -> discrete kalman filter/4(D)
  discrete kalman filter/1(state_est) -> Demux3/1
  discrete kalman filter/2(P_est) -> Unit Delay1/1
  Unit Delay1/1 -> discrete kalman filter/9(P)
  yaw_rate_cmd/1 -> discrete kalman filter/7(u)
  Mux4/1 -> Unit Delay External IC1/2, discrete kalman filter/8(y)
  Q/1 -> discrete kalman filter/5(Q)
  R/1 -> discrete kalman filter/6(R)
  Demux3/2 -> Saturation/1
  Demux3/1 -> Unit Delay External IC1/1, yaw_states_est/1
  Saturation/1 -> yaw_rate_bias/1
  Mux1/1 -> discrete kalman filter/10(state)
  yaw_rate_bias_in/1 -> Mux1/2
  Unit Delay External IC1/1 -> Mux1/1

== system Hquad_control_LIB_MPC/z controller MPC FG ==
  reset : Inport  PortDimensions=1
  X_ref_z : Inport  Port=2
  "z_states_est  " : Inport  Port=3
  AA_delay : Constant  Value=FG_ctrl_z.AA_delay
  BB_delay : Constant  Value=FG_ctrl_z.BB_delay
  L : Constant  Value=FG_ctrl_z.L
  LL_PP : Constant  Value=FG_ctrl_z.LL_PP
  LL_U_ref_PP : Constant  Value=FG_ctrl_z.LL_U_ref_PP
  LL_ref_PP : Constant  Value=FG_ctrl_z.LL_ref_PP
  MM : Constant  Value=FG_ctrl_z.MM
  PP : Constant  Value=FG_ctrl_z.PP
  TT_PP : Constant  Value=FG_ctrl_z.TT_PP
  Unit Delay : UnitDelay  X0=zeros(FG_ctrl_z.delay_steps,1)  SampleTime=-1
  Unit Delay1 : UnitDelay  X0=zeros(size(FG_ctrl_z.V_max,1),1)  SampleTime=-1
  V_max : Constant  Value=FG_ctrl_z.V_max
  betas : Constant  Value=FG_ctrl_z.betas
  i_min : Constant  Value=FG_ctrl_z.i_min
  runFastGradient : MATLAB Function  TreatAsAtomicUnit=on
  thrust_cmd : Outport  PortDimensions=1
  wires:
  "z_states_est  "/1 -> runFastGradient/9(x)
  runFastGradient/1(u_opt) -> thrust_cmd/1
  X_ref_z/1 -> runFastGradient/10(X_ref)
  TT_PP/1 -> runFastGradient/1(TT_PP)
  LL_PP/1 -> runFastGradient/2(LL_PP)
  runFastGradient/4(V_init_out) -> Unit Delay1/1
  runFastGradient/3(u_buff_out) -> Unit Delay/1
  Unit Delay1/1 -> runFastGradient/16(V_init)
  Unit Delay/1 -> runFastGradient/15(u_buff)
  LL_ref_PP/1 -> runFastGradient/3(LL_ref_PP)
  MM/1 -> runFastGradient/5(MM)
  PP/1 -> runFastGradient/6(PP)
  AA_delay/1 -> runFastGradient/7(AA_delay)
  BB_delay/1 -> runFastGradient/8(BB_delay)
  V_max/1 -> runFastGradient/11(V_max)
  i_min/1 -> runFastGradient/12(i_min)
  betas/1 -> runFastGradient/13(betas)
  L/1 -> runFastGradient/14(L)
  LL_U_ref_PP/1 -> runFastGradient/4(LL_U_ref_PP)

== system Hquad_control_LIB_MPC/z states estimator bias ==
  thrust_cmd : Inport  PortDimensions=1
  z_states_meas : Inport  Port=2  PortDimensions=2
  thrust_bias_in : Inport  Port=3  PortDimensions=1
  A : Constant  Value=kalm_mpc_z.A
  B : Constant  Value=kalm_mpc_z.B
  Bus Selector3 : BusSelector  OutputSignals=z,z_dot
  C : Constant  Value=kalm_mpc_z.C
  D : Constant  Value=kalm_mpc_z.D
  Demux3 : Demux  Outputs=2
  Mux1 : Mux  Inputs=2
  Mux4 : Mux  Inputs=2
  Q : Constant  Value=kalm_mpc_z.Q
  R : Constant  Value=kalm_mpc_z.R
  Saturation : Saturate  UpperLimit=MAX_BIAS_THRUST  LowerLimit=-MAX_BIAS_THRUST
  Unit Delay External IC1 : simulink/Additional Math & Discrete/Additional Discrete/Unit Delay External IC  SystemSampleTime=-1  tsamp=-1
  Unit Delay1 : UnitDelay  X0=kalm_mpc_z.P  SampleTime=Ts
  discrete kalman filter : MATLAB Function  AncestorBlock=Hquad_control_LIB_LQRI/x states estimator/discrete kalman filter  TreatAsAtomicUnit=on
  z_states_est : Outport  PortDimensions=2
  thrust_bias : Outport  Port=2  PortDimensions=1
  wires:
  Unit Delay External IC1/1 -> Mux1/1
  thrust_bias_in/1 -> Mux1/2
  Mux1/1 -> discrete kalman filter/10(state)
  Saturation/1 -> thrust_bias/1
  Demux3/1 -> z_states_est/1, Unit Delay External IC1/1
  Demux3/2 -> Saturation/1
  R/1 -> discrete kalman filter/6(R)
  Q/1 -> discrete kalman filter/5(Q)
  Mux4/1 -> discrete kalman filter/8(y), Unit Delay External IC1/2
  thrust_cmd/1 -> discrete kalman filter/7(u)
  Unit Delay1/1 -> discrete kalman filter/9(P)
  discrete kalman filter/2(P_est) -> Unit Delay1/1
  discrete kalman filter/1(state_est) -> Demux3/1
  D/1 -> discrete kalman filter/4(D)
  C/1 -> discrete kalman filter/3(C)
  B/1 -> discrete kalman filter/2(B)
  A/1 -> discrete kalman filter/1(A)
  z_states_meas/1 -> Bus Selector3/1
  Bus Selector3/1 -> Mux4/1  "<z>"
  Bus Selector3/2 -> Mux4/2  "<z_dot>"

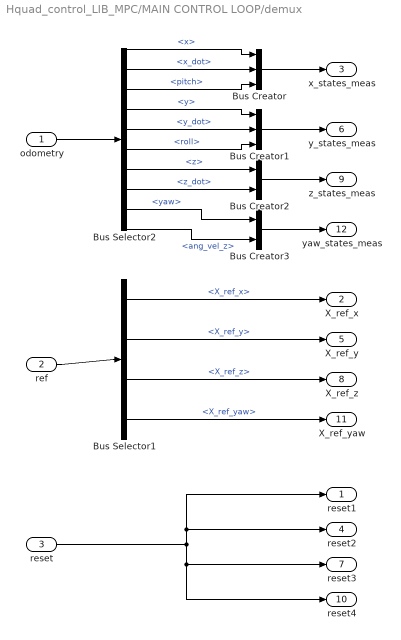
== system Hquad_control_LIB_MPC/MAIN CONTROL LOOP/demux ==
  odometry : Inport
  ref : Inport  Port=2
  reset : Inport  Port=3
  Bus Creator : BusCreator  Inputs=3
  Bus Creator1 : BusCreator  Inputs=3
  Bus Creator2 : BusCreator  Inputs=2
  Bus Creator3 : BusCreator  Inputs=2
  Bus Selector1 : BusSelector  OutputSignals=X_ref_x,X_ref_y,X_ref_z,X_ref_yaw
  Bus Selector2 : BusSelector  OutputSignals=pos.x,vel.x_dot,rpy.pitch,pos.y,vel.y_dot,rpy.roll,pos.z,vel.z_dot,rpy.yaw,ang_vel.ang_vel_z
  reset1 : Outport
  X_ref_x : Outport  Port=2
  x_states_meas : Outport  Port=3  PortDimensions=3
  reset2 : Outport  Port=4
  X_ref_y : Outport  Port=5
  y_states_meas : Outport  Port=6  PortDimensions=3
  reset3 : Outport  Port=7
  X_ref_z : Outport  Port=8
  z_states_meas : Outport  Port=9  PortDimensions=2
  reset4 : Outport  Port=10
  X_ref_yaw : Outport  Port=11
  yaw_states_meas : Outport  Port=12  PortDimensions=2
  wires:
  reset/1 -> reset1/1, reset2/1, reset4/1, reset3/1
  Bus Selector1/2 -> X_ref_y/1  "<X_ref_y>"
  Bus Selector1/1 -> X_ref_x/1  "<X_ref_x>"
  ref/1 -> Bus Selector1/1
  Bus Creator3/1 -> yaw_states_meas/1
  Bus Creator2/1 -> z_states_meas/1
  Bus Selector2/10 -> Bus Creator3/2  "<ang_vel_z>"
  Bus Selector2/9 -> Bus Creator3/1  "<yaw>"
  Bus Selector2/8 -> Bus Creator2/2  "<z_dot>"
  Bus Selector2/7 -> Bus Creator2/1  "<z>"
  Bus Creator1/1 -> y_states_meas/1
  Bus Selector2/5 -> Bus Creator1/2  "<y_dot>"
  Bus Selector2/4 -> Bus Creator1/1  "<y>"
  Bus Selector2/2 -> Bus Creator/2  "<x_dot>"
  Bus Selector2/1 -> Bus Creator/1  "<x>"
  Bus Creator/1 -> x_states_meas/1
  odometry/1 -> Bus Selector2/1
  Bus Selector2/3 -> Bus Creator/3  "<pitch>"
  Bus Selector2/6 -> Bus Creator1/3  "<roll>"
  Bus Selector1/3 -> X_ref_z/1  "<X_ref_z>"
  Bus Selector1/4 -> X_ref_yaw/1  "<X_ref_yaw>"

== system Hquad_control_LIB_MPC/decoupling and rotation/decoupling  ==
  "roll_meas  " : Inport  PortDimensions=1
  "pitch_meas  " : Inport  Port=2  PortDimensions=1
  cmd : Inport  Port=3
  mass : Inport  Port=4
  Bus Creator : BusCreator
  Bus Selector3 : BusSelector  OutputSignals=pitch_cmd,roll_cmd,thrust_cmd,yaw_rate_cmd
  Embedded MATLAB Function : MATLAB Function  TreatAsAtomicUnit=on
  g : Constant  Value=g
  "cmd_comp  " : Outport
  wires:
  g/1 -> Embedded MATLAB Function/7(g)
  mass/1 -> Embedded MATLAB Function/6(m)
  Bus Selector3/3 -> Embedded MATLAB Function/5(thrust)  "<thrust_cmd>"
  Bus Selector3/2 -> Embedded MATLAB Function/4(roll_cmd)  "<roll_cmd>"
  Bus Selector3/1 -> Embedded MATLAB Function/3(pitch_cmd)  "<pitch_cmd>"
  Embedded MATLAB Function/1(pitch_cmd_comp) -> Bus Creator/1  "pitch_cmd"
  Embedded MATLAB Function/2(roll_cmd_comp) -> Bus Creator/2  "roll_cmd"
  Embedded MATLAB Function/3(thrust_comp) -> Bus Creator/3  "thrust_cmd"
  Bus Creator/1 -> "cmd_comp  "/1
  Bus Selector3/4 -> Bus Creator/4  "<yaw_rate_cmd>"
  cmd/1 -> Bus Selector3/1
  "pitch_meas  "/1 -> Embedded MATLAB Function/1(pitch_meas)
  "roll_meas  "/1 -> Embedded MATLAB Function/2(roll_meas)

== system Hquad_control_LIB_MPC/decoupling and rotation/rotate_to_quat_frame ==
  yaw_meas : Inport
  cmd_comp : Inport  Port=2
  bias : Inport  Port=3
  Bus Creator1 : BusCreator
  Bus Creator2 : BusCreator
  Bus Selector1 : BusSelector  OutputSignals=thrust_bias,yaw_rate_bias
  Bus Selector2 : BusSelector  OutputSignals=pitch_bias,roll_bias
  Bus Selector3 : BusSelector  OutputSignals=pitch_cmd,roll_cmd
  Bus Selector4 : BusSelector  OutputSignals=thrust_cmd,yaw_rate_cmd
  Embedded MATLAB Function : MATLAB Function  TreatAsAtomicUnit=on
  "cmd_rot  " : Outport
  bias_rot : Outport  Port=2
  wires:
  Bus Selector1/2 -> Bus Creator1/4  "<yaw_rate_bias>"
  Bus Selector1/1 -> Bus Creator1/3  "<thrust_bias>"
  Bus Selector4/2 -> Bus Creator2/4  "<yaw_rate_cmd>"
  Bus Selector4/1 -> Bus Creator2/3  "<thrust_cmd>"
  Embedded MATLAB Function/2(roll_rot) -> Bus Creator2/2  "roll_cmd"
  Embedded MATLAB Function/1(pitch_rot) -> Bus Creator2/1  "pitch_cmd"
  cmd_comp/1 -> Bus Selector4/1, Bus Selector3/1
  Bus Selector3/1 -> Embedded MATLAB Function/2(pitch_cmd)  "<pitch_cmd>"
  Bus Selector3/2 -> Embedded MATLAB Function/3(roll_cmd)  "<roll_cmd>"
  Bus Creator2/1 -> "cmd_rot  "/1
  Embedded MATLAB Function/4(roll_bias_rot) -> Bus Creator1/2  "roll_bias"
  Embedded MATLAB Function/3(pitch_bias_rot) -> Bus Creator1/1  "pitch_bias"
  Bus Selector2/2 -> Embedded MATLAB Function/5(roll_bias)  "<roll_bias>"
  Bus Selector2/1 -> Embedded MATLAB Function/4(pitch_bias)  "<pitch_bias>"
  Bus Creator1/1 -> bias_rot/1
  bias/1 -> Bus Selector1/1, Bus Selector2/1
  yaw_meas/1 -> Embedded MATLAB Function/1(yaw)

== system Hquad_control_LIB_MPC/pos controller/get ref from vector ==
  X_ref : Inport
  Bus Creator2 : BusCreator
  Bus Creator3 : BusCreator
  Bus Creator4 : BusCreator  Inputs=2
  Bus Selector : BusSelector  OutputSignals=X_ref_x,X_ref_y,X_ref_z,X_ref_yaw
  Demux{1..4} (4 alike) : Demux  Outputs=2
  Selector{,1..3} (4 alike) : Selector  IndexOptions=Index vector (dialog)  Indices=[1 2]  OutputSizes=1
  ref : Outport
  wires:
  Demux4/2 -> Bus Creator3/4  "yaw_dot_ref"
  Demux3/2 -> Bus Creator3/3  "z_dot_ref"
  Demux2/2 -> Bus Creator3/2  "y_dot_ref"
  Demux1/2 -> Bus Creator3/1  "x_dot_ref"
  Demux4/1 -> Bus Creator2/4  "yaw_ref"
  Demux3/1 -> Bus Creator2/3  "z_ref"
  Demux2/1 -> Bus Creator2/2  "y_ref"
  Demux1/1 -> Bus Creator2/1  "x_ref"
  Bus Creator4/1 -> ref/1  "ref"
  Bus Creator3/1 -> Bus Creator4/2  "vel_ref"
  Bus Creator2/1 -> Bus Creator4/1  "pose_ref"
  Selector1/1 -> Demux2/1
  Selector2/1 -> Demux3/1
  Selector3/1 -> Demux4/1
  Selector/1 -> Demux1/1
  Bus Selector/2 -> Selector1/1  "<X_ref_y>"
  Bus Selector/3 -> Selector2/1  "<X_ref_z>"
  Bus Selector/4 -> Selector3/1  "<X_ref_yaw>"
  Bus Selector/1 -> Selector/1  "<X_ref_x>"
  X_ref/1 -> Bus Selector/1

== system Hquad_control_LIB_MPC/traj controller/get ref from vector ==
  X_ref : Inport
  Bus Creator2 : BusCreator
  Bus Creator3 : BusCreator
  Bus Creator4 : BusCreator  Inputs=2
  Bus Selector : BusSelector  OutputSignals=X_ref_x,X_ref_y,X_ref_z,X_ref_yaw
  Demux{1..4} (4 alike) : Demux  Outputs=2
  Selector{,1..3} (4 alike) : Selector  IndexOptions=Index vector (dialog)  Indices=[1 2]  OutputSizes=1
  ref : Outport
  wires:
  Demux4/2 -> Bus Creator3/4  "yaw_dot_ref"
  Demux3/2 -> Bus Creator3/3  "z_dot_ref"
  Demux2/2 -> Bus Creator3/2  "y_dot_ref"
  Demux1/2 -> Bus Creator3/1  "x_dot_ref"
  Demux4/1 -> Bus Creator2/4  "yaw_ref"
  Demux3/1 -> Bus Creator2/3  "z_ref"
  Demux2/1 -> Bus Creator2/2  "y_ref"
  Demux1/1 -> Bus Creator2/1  "x_ref"
  Bus Creator4/1 -> ref/1  "ref"
  Bus Creator3/1 -> Bus Creator4/2  "vel_ref"
  Bus Creator2/1 -> Bus Creator4/1  "pose_ref"
  Selector1/1 -> Demux2/1
  Selector2/1 -> Demux3/1
  Selector3/1 -> Demux4/1
  Selector/1 -> Demux1/1
  Bus Selector/2 -> Selector1/1  "<X_ref_y>"
  Bus Selector/3 -> Selector2/1  "<X_ref_z>"
  Bus Selector/4 -> Selector3/1  "<X_ref_yaw>"
  Bus Selector/1 -> Selector/1  "<X_ref_x>"
  X_ref/1 -> Bus Selector/1

== matlab function decoupling and rotation/decoupling /Embedded MATLAB Function ==
  data: pitch_cmd_comp output double; roll_cmd_comp output double; pitch_meas input double; thrust_comp output double; roll_meas input double; pitch_cmd input double; roll_cmd input double; thrust input double; m input double; g input double
function [pitch_cmd_comp, roll_cmd_comp, thrust_comp]  = fcn(pitch_meas, roll_meas, pitch_cmd, roll_cmd, thrust,m,g)
%#eml

thrust_comp=thrust/(cos(pitch_meas)*cos(roll_meas));

pitch_cmd_comp = m*g/thrust_comp*pitch_cmd;
roll_cmd_comp = m*g/thrust_comp*roll_cmd;

% pitch_cmd_comp=pitch_cmd;
% roll_cmd_comp=roll_cmd;
% pitch_cmd_comp = atan(Fx/(-thrust_comp));
% roll_cmd_comp = atan(Fy/(thrust_comp));

% pitch_cmd_comp = atan(-g*m*pitch_cmd/(-thrust));
% roll_cmd_comp = atan(g*m*roll_cmd*cos(pitch_meas)/(thrust));

== matlab function create ref traj/generate_X_ref_x ==
  data: traj_x input double; X_ref_x output double; idx input double
function X_ref_x  = fcn(traj_x,idx)

pred_horizon_x=30;

X_ref_x=traj_x(:,idx:idx+pred_horizon_x);

== matlab function y states estimator bias/discrete kalman filter ==
  data: A input double; B input double; state_est output double; C input double; D input double; Q input double; R input double; u input double; y input double; P input double; state input double; P_est output double
function [state_est,P_est]  = fcn(A,B,C,D,Q,R, u, y, P, state)
%#eml

% Kalman filter according to Welch & Bishop, An Introduction to the Kalman
% Filter

n=size(A,1);

% Time update
x_=A*state+B*u;
P_=A*P*A'+Q;
  
% Measurement update
K=P_*C'*(C*P_*C'+R)^-1;
state_est=x_+K*(y-C*x_);
P_est=(eye(n)-K*C)*P_;

== matlab function decoupling and rotation/rotate_to_quat_frame/Embedded MATLAB Function ==
  data: yaw input double; pitch_rot output double; pitch_cmd input double; roll_cmd input double; pitch_bias input double; roll_bias input double; roll_rot output double; pitch_bias_rot output double; roll_bias_rot output double
function [pitch_rot,roll_rot, pitch_bias_rot,roll_bias_rot] = fcn(yaw, pitch_cmd, roll_cmd, pitch_bias, roll_bias)

sin_yaw=sin(yaw);
cos_yaw=cos(yaw);

R=[cos_yaw, sin_yaw; -sin_yaw, cos_yaw];

temp=R'*[pitch_cmd;roll_cmd];
pitch_rot=temp(1);
roll_rot=temp(2);

temp=R'*[pitch_bias;roll_bias];
pitch_bias_rot=temp(1);
roll_bias_rot=temp(2);

== matlab function yaw states estimator bias/discrete kalman filter ==
  data: A input double; B input double; state_est output double; C input double; D input double; Q input double; R input double; u input double; y input double; P input double; state input double; P_est output double
function [state_est,P_est]  = fcn(A,B,C,D,Q,R, u, y, P, state)
%#eml

% Kalman filter according to Welch & Bishop, An Introduction to the Kalman
% Filter

n=size(A,1);

% Time update
x_=A*state+B*u;
P_=A*P*A'+Q;
  
% Measurement update
K=P_*C'*(C*P_*C'+R)^-1;
state_est=x_+K*(y-C*x_);
P_est=(eye(n)-K*C)*P_;

== matlab function x controller MPC FG /runFastGradient ==
  data: TT_PP input double; u_opt output double; LL_PP input double; LL_ref_PP input double; LL_U_ref_PP input double; J_star output double; u_buff_out output double; V_init_out output double; MM input double; PP input double; AA_delay input double; BB_delay input double; x input double; X_ref input double; V_max input double; i_min input double; betas input double; L input double; u_buff input double; V_init input double
function [u_opt, J_star, u_buff_out, V_init_out] = fcn(TT_PP, LL_PP,...    
                        LL_ref_PP,LL_U_ref_PP, MM, PP, AA_delay, BB_delay, x, X_ref,...
                        V_max,i_min, betas, L, u_buff, V_init)

    % ugly, but simulink needs fix output sizes for vectors
    m = size(V_max,2); % number of outputs u
    delay_steps = size(BB_delay,2); % number of delay steps
    N = size(V_max,1); % prediction horizon
    
    % predict non-delayed state
    if(delay_steps==0)
        x_predicted=x;
    else
        x_predicted=AA_delay*x+BB_delay*u_buff;
    end
    
    % TODO get U_ref from trajectory
    U_ref=zeros(N,1);
    
    % set optimization variables
    LL_PP_ref=x_predicted'*LL_PP - X_ref'*LL_ref_PP - U_ref' * LL_U_ref_PP;
    MM_ref = x_predicted' * MM * x_predicted; % TODO expand to X_ref, U_ref
    
    % run fast gradient method
    [J_star, V_star, ~] = ...
        runFastGradient(TT_PP, LL_PP_ref, MM_ref, -V_max, V_max, V_init, ...
        i_min, betas, L, []);
    
    
    % Note: Fast gradient method is implemented in variable V where U = PP * V,
    % so don't forget to backtransform after termination:
    U_star = PP * V_star;

     % save outputs for delayed system
    if(delay_steps==0)
        u_buff_out=0;
    else
        u_buff_out=[u_buff(2:delay_steps,:); U_star(1:m,1)];
    end
 
    % set new initial guess
    V_init_out=[V_star(2:N);0];
    
    u_opt=U_star(1:m,1);

== matlab function y controller MPC FG/runFastGradient ==
  data: TT_PP input double; u_opt output double; LL_PP input double; LL_ref_PP input double; LL_U_ref_PP input double; J_star output double; u_buff_out output double; V_init_out output double; MM input double; PP input double; AA_delay input double; BB_delay input double; x input double; X_ref input double; V_max input double; i_min input double; betas input double; L input double; u_buff input double; V_init input double
function [u_opt, J_star, u_buff_out, V_init_out] = fcn(TT_PP, LL_PP,...    
                        LL_ref_PP,LL_U_ref_PP, MM, PP, AA_delay, BB_delay, x, X_ref,...
                        V_max,i_min, betas, L, u_buff, V_init)

    % ugly, but simulink needs fix output sizes for vectors
    m = size(V_max,2); % number of outputs u
    delay_steps = size(BB_delay,2); % number of delay steps
    N = size(V_max,1); % prediction horizon
    
    % predict non-delayed state
    if(delay_steps==0)
        x_predicted=x;
    else
        x_predicted=AA_delay*x+BB_delay*u_buff;
    end
    
    % TODO get U_ref from trajectory
    U_ref=zeros(N,1);
    
    % set optimization variables
    LL_PP_ref=x_predicted'*LL_PP - X_ref'*LL_ref_PP - U_ref' * LL_U_ref_PP;
    MM_ref = x_predicted' * MM * x_predicted; % TODO expand to X_ref, U_ref
    
    % run fast gradient method
    [J_star, V_star, ~] = ...
        runFastGradient(TT_PP, LL_PP_ref, MM_ref, -V_max, V_max, V_init, ...
        i_min, betas, L, []);
    
    
    % Note: Fast gradient method is implemented in variable V where U = PP * V,
    % so don't forget to backtransform after termination:
    U_star = PP * V_star;

     % save outputs for delayed system
    if(delay_steps==0)
        u_buff_out=0;
    else
        u_buff_out=[u_buff(2:delay_steps,:); U_star(1:m,1)];
    end
 
    % set new initial guess
    V_init_out=[V_star(2:N);0];
    
    u_opt=U_star(1:m,1);
